simulink model "ExampleTrafficLights_2KFlatLHD"  (Simulink 9.2)
settings: Solver=FixedStepDiscrete  StartTime=0.0  StopTime=Inf  FixedStep=0.001  RelTol=1e-3  EnableMultiTasking=on
libraries: rFproPhysicsLib x40
settings Model: Creator=SeanK  LastModifiedBy=SeanKavanagh
settings DataIOCC: SignalLoggingSaveFormat=Dataset
settings DebuggingCC: SolverPrmCheckMsg=warning  FcnCallInpInsideContextMsg=error  StateNameClashWarn=none
settings RTWCC: SystemTargetFile=rfpro.tlc  MakeCommand="make_rtw OPTS=\"-DRUN_PHYSICS\""  TemplateMakefile=rfpro.tmf  Description=rFpro Target (Run Physics)  TargetLang=C++
settings STFCustomTargetCC: ModelReferenceCompliant=off  GeneratePreprocessorConditionals=Disable all  CombineOutputUpdateFcns=on  MatFileLogging=on  CPPClassGenCompliant=on  GRTInterface=off  SystemTargetFile=rfpro.tlc
settings GRTTargetCC: ModelReferenceCompliant=off  ParMdlRefBuildCompliant=off  CompOptLevelCompliant=off  ConcurrentExecutionCompliant=off  CombineOutputUpdateFcns=on  GRTInterface=off  UseToolchainInfoCompliant=off

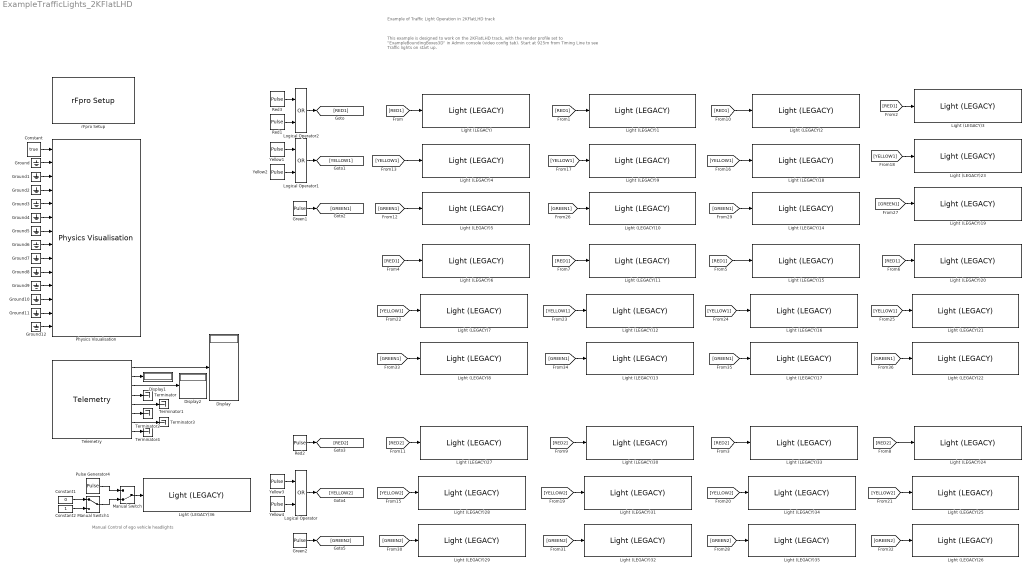
== system ExampleTrafficLights_2KFlatLHD ==
  note: This example is designed to work on the 2KFlatLHD track,
      | with the render profile set to "ExampleBoundingBoxes3D" in Admin console (video config tab).
      |
      | Start at 925m from Timing Line to see Traffic lights on start up.
  note: Manual Control of ego vehicle headlights
  note: Example of Traffic Light Operation in 2KFlatLHD track
  Constant : Constant  Value=true
  Constant1 : Constant  Value=0
  Constant2 : Constant
  Display : Display
  Display1 : Display
  Display2 : Display
  Green1 : DiscretePulseGenerator  PulseType=Time based  Period=8  PulseWidth=25  PhaseDelay=4
  Green2 : DiscretePulseGenerator  PulseType=Time based  Period=8  PulseWidth=25
  Ground{,1..12} (13 alike) : Ground
  Light (LEGACY) : rFproPhysicsLib/Legacy Blocks/Light (LEGACY)  light_name='TL_01_01_STD_R'  exact_match=on  on_vehicle=off  useReverseByteOrder=off  rFpro__platform=Remote Model - Default
  Light (LEGACY)1 : rFproPhysicsLib/Legacy Blocks/Light (LEGACY)  light_name='TL_01_02_STD_R'  exact_match=on  on_vehicle=off  useReverseByteOrder=off  rFpro__platform=Remote Model - Default
  Light (LEGACY)10 : rFproPhysicsLib/Legacy Blocks/Light (LEGACY)  light_name='TL_01_02_STD_G'  exact_match=on  on_vehicle=off  useReverseByteOrder=off  rFpro__platform=Remote Model - Default
  Light (LEGACY)11 : rFproPhysicsLib/Legacy Blocks/Light (LEGACY)  light_name='TL_01_10_STD_R'  exact_match=on  on_vehicle=off  useReverseByteOrder=off  rFpro__platform=Remote Model - Default
  Light (LEGACY)12 : rFproPhysicsLib/Legacy Blocks/Light (LEGACY)  light_name='TL_01_10_STD_Y'  exact_match=on  on_vehicle=off  useReverseByteOrder=off  rFpro__platform=Remote Model - Default
  Light (LEGACY)13 : rFproPhysicsLib/Legacy Blocks/Light (LEGACY)  light_name='TL_01_10_STD_G'  exact_match=on  on_vehicle=off  useReverseByteOrder=off  rFpro__platform=Remote Model - Default
  Light (LEGACY)14 : rFproPhysicsLib/Legacy Blocks/Light (LEGACY)  light_name='TL_01_03_STD_G'  exact_match=on  on_vehicle=off  useReverseByteOrder=off  rFpro__platform=Remote Model - Default
  Light (LEGACY)15 : rFproPhysicsLib/Legacy Blocks/Light (LEGACY)  light_name='TL_01_11_STD_R'  exact_match=on  on_vehicle=off  useReverseByteOrder=off  rFpro__platform=Remote Model - Default
  Light (LEGACY)16 : rFproPhysicsLib/Legacy Blocks/Light (LEGACY)  light_name='TL_01_11_STD_Y'  exact_match=on  on_vehicle=off  useReverseByteOrder=off  rFpro__platform=Remote Model - Default
  Light (LEGACY)17 : rFproPhysicsLib/Legacy Blocks/Light (LEGACY)  light_name='TL_01_11_STD_G'  exact_match=on  on_vehicle=off  useReverseByteOrder=off  rFpro__platform=Remote Model - Default
  Light (LEGACY)18 : rFproPhysicsLib/Legacy Blocks/Light (LEGACY)  light_name='TL_01_03_STD_Y'  exact_match=on  on_vehicle=off  useReverseByteOrder=off  rFpro__platform=Remote Model - Default
  Light (LEGACY)19 : rFproPhysicsLib/Legacy Blocks/Light (LEGACY)  light_name='TL_01_04_STD_G'  exact_match=on  on_vehicle=off  useReverseByteOrder=off  rFpro__platform=Remote Model - Default
  Light (LEGACY)2 : rFproPhysicsLib/Legacy Blocks/Light (LEGACY)  light_name='TL_01_03_STD_R'  exact_match=on  on_vehicle=off  useReverseByteOrder=off  rFpro__platform=Remote Model - Default
  Light (LEGACY)20 : rFproPhysicsLib/Legacy Blocks/Light (LEGACY)  light_name='TL_01_12_STD_R'  exact_match=on  on_vehicle=off  useReverseByteOrder=off  rFpro__platform=Remote Model - Default
  Light (LEGACY)21 : rFproPhysicsLib/Legacy Blocks/Light (LEGACY)  light_name='TL_01_12_STD_Y'  exact_match=on  on_vehicle=off  useReverseByteOrder=off  rFpro__platform=Remote Model - Default
  Light (LEGACY)22 : rFproPhysicsLib/Legacy Blocks/Light (LEGACY)  light_name='TL_01_12_STD_G'  exact_match=on  on_vehicle=off  useReverseByteOrder=off  rFpro__platform=Remote Model - Default
  Light (LEGACY)23 : rFproPhysicsLib/Legacy Blocks/Light (LEGACY)  light_name='TL_01_04_STD_Y'  exact_match=on  on_vehicle=off  useReverseByteOrder=off  rFpro__platform=Remote Model - Default
  Light (LEGACY)24 : rFproPhysicsLib/Legacy Blocks/Light (LEGACY)  light_name='TL_01_08_STD_R'  exact_match=on  on_vehicle=off  useReverseByteOrder=off  rFpro__platform=Remote Model - Default
  Light (LEGACY)25 : rFproPhysicsLib/Legacy Blocks/Light (LEGACY)  light_name='TL_01_08_STD_Y'  exact_match=on  on_vehicle=off  useReverseByteOrder=off  rFpro__platform=Remote Model - Default
  Light (LEGACY)26 : rFproPhysicsLib/Legacy Blocks/Light (LEGACY)  light_name='TL_01_08_STD_G'  exact_match=on  on_vehicle=off  useReverseByteOrder=off  rFpro__platform=Remote Model - Default
  Light (LEGACY)27 : rFproPhysicsLib/Legacy Blocks/Light (LEGACY)  light_name='TL_01_05_STD_R'  exact_match=on  on_vehicle=off  useReverseByteOrder=off  rFpro__platform=Remote Model - Default
  Light (LEGACY)28 : rFproPhysicsLib/Legacy Blocks/Light (LEGACY)  light_name='TL_01_05_STD_Y'  exact_match=on  on_vehicle=off  useReverseByteOrder=off  rFpro__platform=Remote Model - Default
  Light (LEGACY)29 : rFproPhysicsLib/Legacy Blocks/Light (LEGACY)  light_name='TL_01_05_STD_G'  exact_match=on  on_vehicle=off  useReverseByteOrder=off  rFpro__platform=Remote Model - Default
  Light (LEGACY)3 : rFproPhysicsLib/Legacy Blocks/Light (LEGACY)  light_name='TL_01_04_STD_R'  exact_match=on  on_vehicle=off  useReverseByteOrder=off  rFpro__platform=Remote Model - Default
  Light (LEGACY)30 : rFproPhysicsLib/Legacy Blocks/Light (LEGACY)  light_name='TL_01_06_STD_R'  exact_match=on  on_vehicle=off  useReverseByteOrder=off  rFpro__platform=Remote Model - Default
  Light (LEGACY)31 : rFproPhysicsLib/Legacy Blocks/Light (LEGACY)  light_name='TL_01_06_STD_Y'  exact_match=on  on_vehicle=off  useReverseByteOrder=off  rFpro__platform=Remote Model - Default
  Light (LEGACY)32 : rFproPhysicsLib/Legacy Blocks/Light (LEGACY)  light_name='TL_01_06_STD_G'  exact_match=on  on_vehicle=off  useReverseByteOrder=off  rFpro__platform=Remote Model - Default
  Light (LEGACY)33 : rFproPhysicsLib/Legacy Blocks/Light (LEGACY)  light_name='TL_01_07_STD_R'  exact_match=on  on_vehicle=off  useReverseByteOrder=off  rFpro__platform=Remote Model - Default
  Light (LEGACY)34 : rFproPhysicsLib/Legacy Blocks/Light (LEGACY)  light_name='TL_01_07_STD_Y'  exact_match=on  on_vehicle=off  useReverseByteOrder=off  rFpro__platform=Remote Model - Default
  Light (LEGACY)35 : rFproPhysicsLib/Legacy Blocks/Light (LEGACY)  light_name='TL_01_07_STD_G'  exact_match=on  on_vehicle=off  useReverseByteOrder=off  rFpro__platform=Remote Model - Default
  Light (LEGACY)36 : rFproPhysicsLib/Legacy Blocks/Light (LEGACY)  light_name='HLIGHTDS'  exact_match=on  on_vehicle=on  useReverseByteOrder=off  rFpro__platform=Remote Model - Default
  Light (LEGACY)4 : rFproPhysicsLib/Legacy Blocks/Light (LEGACY)  light_name='TL_01_01_STD_Y'  exact_match=on  on_vehicle=off  useReverseByteOrder=off  rFpro__platform=Remote Model - Default
  Light (LEGACY)5 : rFproPhysicsLib/Legacy Blocks/Light (LEGACY)  light_name='TL_01_01_STD_G'  exact_match=on  on_vehicle=off  useReverseByteOrder=off  rFpro__platform=Remote Model - Default
  Light (LEGACY)6 : rFproPhysicsLib/Legacy Blocks/Light (LEGACY)  light_name='TL_01_09_STD_R'  exact_match=on  on_vehicle=off  useReverseByteOrder=off  rFpro__platform=Remote Model - Default
  Light (LEGACY)7 : rFproPhysicsLib/Legacy Blocks/Light (LEGACY)  light_name='TL_01_09_STD_Y'  exact_match=on  on_vehicle=off  useReverseByteOrder=off  rFpro__platform=Remote Model - Default
  Light (LEGACY)8 : rFproPhysicsLib/Legacy Blocks/Light (LEGACY)  light_name='TL_01_09_STD_G'  exact_match=on  on_vehicle=off  useReverseByteOrder=off  rFpro__platform=Remote Model - Default
  Light (LEGACY)9 : rFproPhysicsLib/Legacy Blocks/Light (LEGACY)  light_name='TL_01_02_STD_Y'  exact_match=on  on_vehicle=off  useReverseByteOrder=off  rFpro__platform=Remote Model - Default
  Logical Operator : Logic  Operator=OR  AllPortsSameDT=off
  Logical Operator1 : Logic  Operator=OR  AllPortsSameDT=off
  Logical Operator2 : Logic  Operator=OR  AllPortsSameDT=off
  Manual Switch : ManualSwitch  CurrentSetting=0
  Manual Switch1 : ManualSwitch
  Physics Visualisation : rFproPhysicsLib/Physics Visualisation  PAR_SKIP_INTERNAL_PHYSICS=off  PAR_ACCEL_VALID=off  PAR_ROT_ACCEL_VALID=off  PAR_GEAR_VALID=off  PAR_RPM_VALID=off  PAR_INPUTS_VALID=on  PAR_STEER_TORQUE_VALID=on  PAR_HEADLIGHTS_ON_VALID=off  PAR_WHEEL_POS_VALID=off  PAR_WHEEL_ORI_VALID=off  PAR_TYRE_PARAMS_VALID=off  PAR_WHEEL_ROTATION_VALID=off  PAR_WHEEL_BRAKE_TEMP_VALID=off  PAR_WHEEL_TREAD_TEMP_VALID=off  PAR_WHEEL_AIR_TEMP_VALID=off  period=-1  offset=0  useReverseByteOrder=on  rFpro__platform=Remote Model - Default
  Pulse Generator4 : DiscretePulseGenerator  PulseType=Time based  PulseWidth=50
  Red1 : DiscretePulseGenerator  PulseType=Time based  Period=8  PulseWidth=100/8  PhaseDelay=7
  Red2 : DiscretePulseGenerator  PulseType=Time based  Period=8  PulseWidth=500/8  PhaseDelay=3
  Red3 : DiscretePulseGenerator  PulseType=Time based  Period=8  PulseWidth=50
  Telemetry : rFproPhysicsLib/Telemetry
  Terminator{,1..4} (5 alike) : Terminator
  Yellow1 : DiscretePulseGenerator  PulseType=Time based  Period=8  PulseWidth=100/8  PhaseDelay=3
  Yellow2 : DiscretePulseGenerator  PulseType=Time based  Period=8  PulseWidth=100/8  PhaseDelay=6
  Yellow3 : DiscretePulseGenerator  PulseType=Time based  Period=8  PulseWidth=100/8  PhaseDelay=2
  Yellow4 : DiscretePulseGenerator  PulseType=Time based  Period=8  PulseWidth=100/8  PhaseDelay=7
  rFpro Setup : rFproPhysicsLib/rFpro Setup  platform=Remote Model - Default  stopOnSessionEnd=on  usePseudoRealtime=on  syncToRF=on  useReverseByteOrder=off  useRfTime=on  minIterations=4  maxIterations=1000  ipReceiveAddress='127.0.0.1'  ipReceivePort=11054  receiveSampleTime=-1  ipTransmitAddress='127.0.0.1'  ipTransmitPort=11052  transmitSampleTime=-1  pluginType=RUN_PHYSICS  sysTarget=xpctarget.tlc  templateMakeFile=xpc_default_tmf  makeCommand=make_rtw  buildDesc=xPC target
  wires:
  Constant/1 -> Physics Visualisation/1
  Ground1/1 -> Physics Visualisation/3
  Ground/1 -> Physics Visualisation/2
  Ground2/1 -> Physics Visualisation/4
  Ground3/1 -> Physics Visualisation/5
  Ground4/1 -> Physics Visualisation/6
  Ground5/1 -> Physics Visualisation/7
  Ground6/1 -> Physics Visualisation/8
  Ground9/1 -> Physics Visualisation/11
  Ground8/1 -> Physics Visualisation/10
  Ground10/1 -> Physics Visualisation/12
  Ground11/1 -> Physics Visualisation/13
  Ground12/1 -> Physics Visualisation/14
  Ground7/1 -> Physics Visualisation/9
  Telemetry/4 -> Terminator/1
  Telemetry/5 -> Terminator1/1
  Telemetry/7 -> Terminator3/1
  Telemetry/6 -> Terminator2/1
  Telemetry/8 -> Terminator4/1
  Telemetry/1 -> Display/1
  Telemetry/2 -> Display1/1
  Telemetry/3 -> Display2/1
  Pulse Generator4/1 -> Manual Switch/1
  Yellow4/1 -> Logical Operator/2
  Yellow3/1 -> Logical Operator/1
  Yellow2/1 -> Logical Operator1/2
  Yellow1/1 -> Logical Operator1/1
  Red1/1 -> Logical Operator2/2
  Red3/1 -> Logical Operator2/1
  Manual Switch/1 -> Light (LEGACY)36/1
  Constant1/1 -> Manual Switch1/1
  Constant2/1 -> Manual Switch1/2
  Manual Switch1/1 -> Manual Switch/2
  Logical Operator2/1 -> [RED1]
  Green1/1 -> [GREEN1]
  Logical Operator1/1 -> [YELLOW1]
  Red2/1 -> [RED2]
  Logical Operator/1 -> [YELLOW2]
  Green2/1 -> [GREEN2]
  [RED1] -> Light (LEGACY)/1
  [RED1] -> Light (LEGACY)1/1
  [RED1] -> Light (LEGACY)2/1
  [RED1] -> Light (LEGACY)3/1
  [YELLOW1] -> Light (LEGACY)4/1
  [GREEN1] -> Light (LEGACY)5/1
  [RED1] -> Light (LEGACY)6/1
  [YELLOW1] -> Light (LEGACY)7/1
  [GREEN1] -> Light (LEGACY)8/1
  [YELLOW1] -> Light (LEGACY)9/1
  [GREEN1] -> Light (LEGACY)10/1
  [RED1] -> Light (LEGACY)11/1
  [YELLOW1] -> Light (LEGACY)12/1
  [GREEN1] -> Light (LEGACY)13/1
  [YELLOW1] -> Light (LEGACY)18/1
  [GREEN1] -> Light (LEGACY)14/1
  [RED1] -> Light (LEGACY)15/1
  [YELLOW1] -> Light (LEGACY)16/1
  [GREEN1] -> Light (LEGACY)17/1
  [YELLOW1] -> Light (LEGACY)23/1
  [GREEN1] -> Light (LEGACY)19/1
  [RED1] -> Light (LEGACY)20/1
  [YELLOW1] -> Light (LEGACY)21/1
  [GREEN1] -> Light (LEGACY)22/1
  [RED2] -> Light (LEGACY)27/1
  [YELLOW2] -> Light (LEGACY)28/1
  [GREEN2] -> Light (LEGACY)29/1
  [RED2] -> Light (LEGACY)30/1
  [YELLOW2] -> Light (LEGACY)31/1
  [GREEN2] -> Light (LEGACY)32/1
  [RED2] -> Light (LEGACY)33/1
  [YELLOW2] -> Light (LEGACY)34/1
  [GREEN2] -> Light (LEGACY)35/1
  [RED2] -> Light (LEGACY)24/1
  [YELLOW2] -> Light (LEGACY)25/1
  [GREEN2] -> Light (LEGACY)26/1
